simulink model "MODEL_SS_withSCCandRL_Emily_Sim_v1"  (R2024b)
settings: Solver=VariableStepAuto  StartTime=0.0  StopTime=80  RelTol=1e-3
PostLoadFcn:
  | Cconst = 0.15915494327;
  | Kp = [76; 141.7; 139.6; 114.2]*Cconst/60;
  | Tp = [14.4; 19.1; 9.39; 9.12];
  | Tg = 0.38*ones(4,1);
  | R = 3/60*ones(4,1);
  | Bagc = [0.416; 0.377; 0.378; 0.388]*60;
  | Kagc = [0.75; 0.25; 0.5; 0.5]*(-0.131);
  | Kdc = ones(4,1);
  | 
  | T = zeros(4,4);
  | T(1, 2) = 0.029;
  | T(1, 3) = 0.0143;
  | T(1, 4) = 0.0099;
  | T(2, 3) = 0.0205;
  | T(3, 4) = 0.0089;
  | T = T.*(60/Cconst);
  | T = T + T';
  | 
  | % State space of system with AGC
  | % x = [Pc Pg w Ptie]
  | % u = [Pl Pdc Pi+1 Pi+2 Pi+3]
  | clear AMatrices BMatrices
  | AMatrices(4) = struct();
  | BMatrices(4) = struct();
  | for i = 1:4
  |     Amatrix = [
  |         0, 0, Kagc(i)*Bagc(i), Kagc(i)
  |         1/Tg(i), -1/Tg(i), -1/Tg(i)/R(i), 0
  |         0, Kp(i), -Tp(i), -Kp(i)
  |         0, 0, sum(T(i,:)), 0
  |     ];
  |     AMatrices(i).value = Amatrix;
  |     Bmatrix = [
  |         0,Kagc(i)*Kdc(i),0,0,0
  |         0,0,0,0,0
  |         -Kp(i),-Kp(i)*Kdc(i),0,0,0
  |         0,0,-T(i, mod(i,4)+1),-T(i, mod(i+1,4)+1),-T(i, mod(i+2,4)+1)
  |     ];
  |     BMatrices(i).value = Bmatrix;
  | end
  | 
  | % Safety Critical Controller system
  | % The input to this system also include the AGC inputs Pc
  | % x = [Pg w Ptie]1,2,3,4
  | % u = [Pc Pl Pdc]1,2,3,4
  | 
  | Ascc = [
  |     AMatrices(1).value(2:4, 2:4), ...
  |     [zeros(3,1), BMatrices(1).value(2:4,3), zeros(3,1)], ...
  |     [zeros(3,1), BMatrices(1).value(2:4,4), zeros(3,1)], ...
  |     [zeros(3,1), BMatrices(1).value(2:4,5), zeros(3,1)]
  | 
  |     [zeros(3,1), BMatrices(2).value(2:4,3), zeros(3,1)], ...
  |     AMatrices(2).value(2:4, 2:4), ...
  |     [zeros(3,1), BMatrices(2).value(2:4,4), zeros(3,1)], ...
  |     [zeros(3,1), BMatrices(2).value(2:4,5), zeros(3,1)]
  | 
  |     [zeros(3,1), BMatrices(3).value(2:4,3), zeros(3,1)], ...
  |     [zeros(3,1), BMatrices(3).value(2:4,4), zeros(3,1)], ...
  |     AMatrices(3).value(2:4, 2:4), ...
  |     [zeros(3,1), BMatrices(3).value(2:4,5), zeros(3,1)]
  | 
  |     [zeros(3,1), BMatrices(4).value(2:4,3), zeros(3,1)], ...
  |     [zeros(3,1), BMatrices(4).value(2:4,4), zeros(3,1)], ...
  |     [zeros(3,1), BMatrices(4).value(2:4,5), zeros(3,1)], ...
  |     AMatrices(4).value(2:4, 2:4)
  | ];
  | 
  | Bscc = [
  |     AMatrices(1).value(2:4, 1), ...
  |     BMatrices(1).value(2:4, 1:2), ...
  |     zeros(3, 9)
  | 
  |     zeros(3,3), ...
  |     AMatrices(2).value(2:4, 1), ...
  |     BMatrices(2).value(2:4, 1:2), ...
  |     zeros(3,6)
  | 
  |     zeros(3,6), ...
  |     AMatrices(3).value(2:4, 1), ...
  |     BMatrices(3).value(2:4, 1:2), ...
  |     zeros(3,3)
  | 
  |     zeros(3,9), ...
  |     AMatrices(4).value(2:4, 1), ...
  |     BMatrices(4).value(2:4, 1:2)
  | ];
  | 
  | C = zeros(4,12);
  | C(1,2) = 1; C(2,5) = 1; C(3,8) = 1; C(4,11) = 1; % extracting the frequencies
libraries: dspsrcs4 x2, rllib x1
settings Model: Creator=amrmo  LastModifiedBy=emily

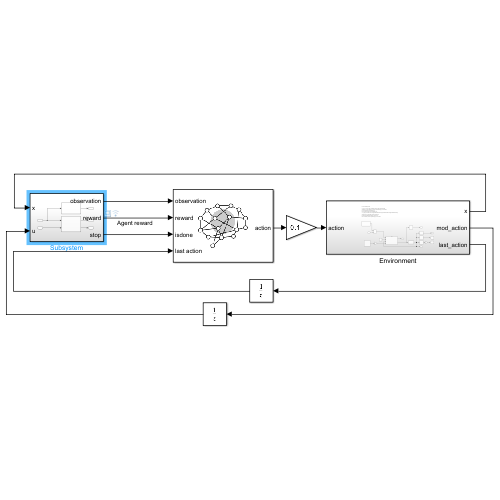
[thumbnail: Simulink's stored preview of the top-level diagram]
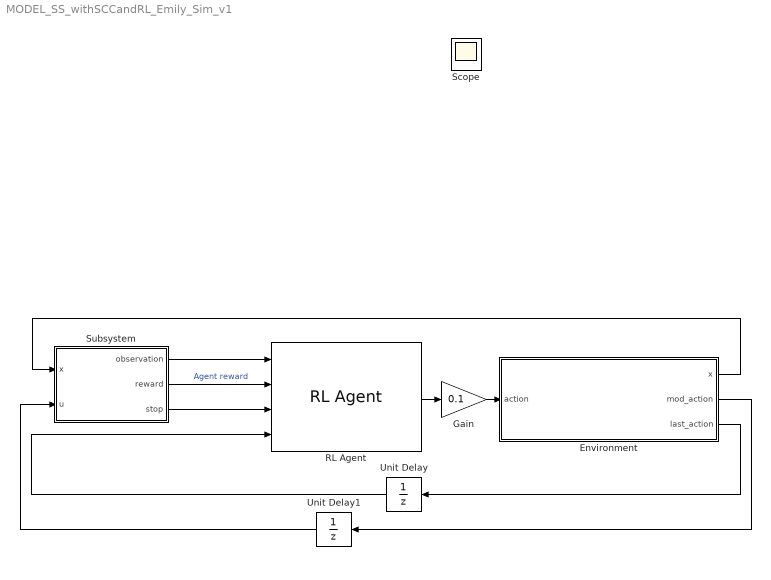
== system MODEL_SS_withSCCandRL_Emily_Sim_v1 ==
  Environment : Subsystem
  Gain : Gain  Gain=0.1
  RL Agent : rllib/RL Agent  Agent=agent  ExternalActionAsInput=off  ProvideLastAction=on  ProvideCumRwd=off  TreatAsDirectFeedthrough=on  UseStrictObservationDataTypes=off
  Subsystem : Subsystem
  Unit Delay : UnitDelay  SampleTime=-1  HasFrameUpgradeWarning=on
  Unit Delay1 : UnitDelay  SampleTime=-1  HasFrameUpgradeWarning=on
  Scope : Scope
  wires:
  RL Agent/1 -> Gain/1
  Environment/3(last_action) -> Unit Delay/1
  Environment/1(x) -> Subsystem/1(x)
  Subsystem/3(stop) -> RL Agent/3
  Subsystem/2(reward) -> RL Agent/2  "Agent reward"
  Subsystem/1(observation) -> RL Agent/1
  Unit Delay/1 -> RL Agent/4
  Gain/1 -> Environment/1(action)
  Environment/2(mod_action) -> Unit Delay1/1
  Unit Delay1/1 -> Subsystem/2(u)

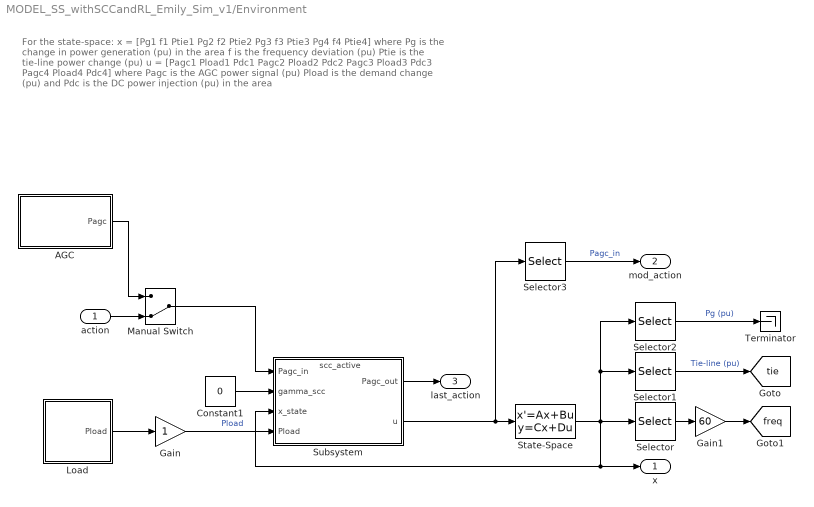
== system MODEL_SS_withSCCandRL_Emily_Sim_v1/Environment ==
  note: For the state-space:
      | x = [Pg1 f1 Ptie1 Pg2 f2 Ptie2 Pg3 f3 Ptie3 Pg4 f4 Ptie4]
      | where Pg is the change in power generation (pu) in the area
      | f is the frequency deviation (pu)
      | Ptie is the tie-line power change (pu)
      | u = [Pagc1 Pload1 Pdc1 Pagc2 Pload2 Pdc2 Pagc3 Pload3 Pdc3 Pagc4 Pload4 Pdc4]
      | where Pagc is the AGC power signal (pu)
      | Pload is the demand change (pu) and
      | Pdc is the DC power injection (pu) in the area
  action : Inport
  AGC : Subsystem
  Constant1 : Constant  Value=0
  Gain : Gain
  Gain1 : Gain  Gain=60
  Load : Subsystem
  Manual Switch : ManualSwitch  CurrentSetting=0
  Selector : Selector  InputPortWidth=12  IndexOptions=Index vector (dialog)  Indices=[2, 5, 8, 11]  OutputSizes=1
  Selector1 : Selector  InputPortWidth=12  IndexOptions=Index vector (dialog)  Indices=[3, 6, 9, 12]  OutputSizes=1
  Selector2 : Selector  InputPortWidth=12  IndexOptions=Index vector (dialog)  Indices=[1, 4, 7, 10]  OutputSizes=1
  Selector3 : Selector  InputPortWidth=12  IndexOptions=Index vector (dialog)  Indices=[1, 4, 7, 10]  OutputSizes=1
  State-Space : StateSpace  A=Ascc  B=Bscc  C=eye(size(Ascc,1))  D=zeros(size(Ascc,1), size(Bscc,2))  InitialCondition=0
  Subsystem : Subsystem
      settings: PortSchema="{\"entries\":[{\"content\":{\"sides\":[{\"content\":{\"connectorIds\":[\"In1\",\"In2\",\"In3\",\"In4\"]},\"type\":\"ConnectorPlacement.EquallySpacedRectSide\",\"uuid\":\"8ad80700-b038-40e4-a204-e695f2c66b8e\"},{\"content\":{\"connectorIds\":[\"Out1\",\"Out2\"],\"side\":\"RIGHT\"},\"type\":\"ConnectorPlacement.EquallySpacedRectSide\",\"uuid\":\"cb352c72-7f98-48f9-8295-4293ff514381\"},{\"content\":{\"connectorIds\":[\"Out3\"],\"side\":\"TOP\"},\"type\":\"ConnectorPlacement.EquallySpacedRectSide\",\"uuid\":\"f93a8a53-617b-4279-a8c2-a1411ef0bdbe\"}]},\"type\":\"ConnectorPlacement.EquallySpacedConnector\",\"uuid\":\"ea4f9763-0230-4afd-86db-2092d4b33ed4\"}],\"packageUris\":[\"http://schema.mathworks.com/mf0/Connector/R2020b\"],\"version\":\"1.0\"}"
  Terminator : Terminator
  x : Outport
  mod_action : Outport  Port=2
  last_action : Outport  Port=3
  tag scope: freq=global, tie=global
  wires:
  Subsystem/2(u) -> Selector3/1, State-Space/1
  Load/1(Pload) -> Gain/1
  Constant1/1 -> Subsystem/2(gamma_scc)
  Gain1/1 -> [freq]
  AGC/1(Pagc) -> Manual Switch/1
  Selector2/1 -> Terminator/1  "Pg (pu)"
  Selector/1 -> Gain1/1
  State-Space/1 -> Selector2/1, Selector1/1, x/1, Subsystem/3(x_state), Selector/1
  Gain/1 -> Subsystem/4(Pload)  "Pload"
  Manual Switch/1 -> Subsystem/1(Pagc_in)
  Selector1/1 -> [tie]  "Tie-line (pu)"
  action/1 -> Manual Switch/2
  Subsystem/1(Pagc_out) -> last_action/1
  Selector3/1 -> mod_action/1  "Pagc_in"

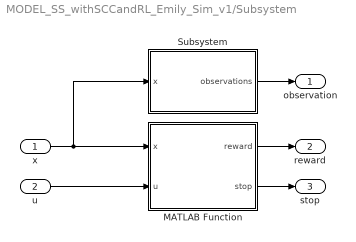
== system MODEL_SS_withSCCandRL_Emily_Sim_v1/Subsystem ==
  x : Inport
  u : Inport  Port=2
  MATLAB Function : MATLAB Function  TreatAsAtomicUnit=on
  Subsystem : Subsystem
  observation : Outport
  reward : Outport  Port=2
  stop : Outport  Port=3
  wires:
  x/1 -> Subsystem/1(x), MATLAB Function/1(x)
  Subsystem/1(observations) -> observation/1
  MATLAB Function/1(reward) -> reward/1
  MATLAB Function/2(stop) -> stop/1
  u/1 -> MATLAB Function/2(u)

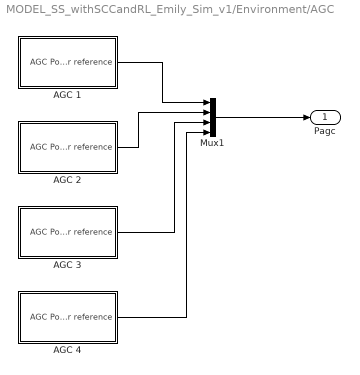
== system MODEL_SS_withSCCandRL_Emily_Sim_v1/Environment/AGC ==
  AGC 1 : Subsystem
  AGC 2 : Subsystem
  AGC 3 : Subsystem
  AGC 4 : Subsystem
  Mux1 : Mux
  Pagc : Outport
  wires:
  AGC 3/1(AGC Power reference) -> Mux1/3
  AGC 4/1(AGC Power reference) -> Mux1/4
  AGC 1/1(AGC Power reference) -> Mux1/1
  AGC 2/1(AGC Power reference) -> Mux1/2
  Mux1/1 -> Pagc/1

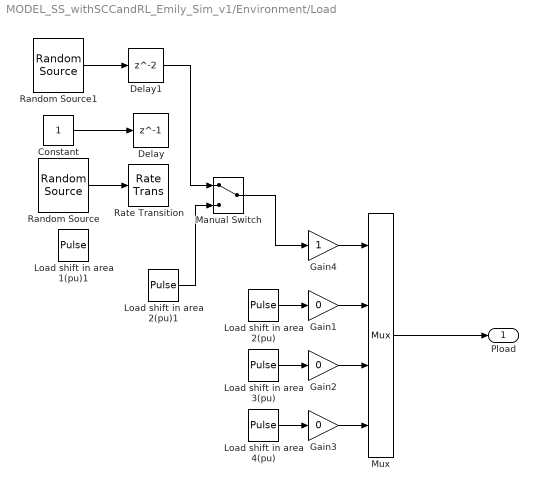
== system MODEL_SS_withSCCandRL_Emily_Sim_v1/Environment/Load ==
  Constant : Constant
  Delay : Delay  DelayLength=1  InitialCondition=0
  Delay1 : Delay  InitialCondition=0
  Gain1 : Gain  Gain=0
  Gain2 : Gain  Gain=0
  Gain3 : Gain  Gain=0
  Gain4 : Gain
  Load shift in area 1(pu)1 : DiscretePulseGenerator  PulseType=Time based  Amplitude=0.05  Period=80  PulseWidth=10  PhaseDelay=10
  Load shift in area 2(pu) : DiscretePulseGenerator  PulseType=Time based  Amplitude=0.2  Period=2*pi/2.5  PulseWidth=40
  Load shift in area 2(pu)1 : DiscretePulseGenerator  PulseType=Time based  Amplitude=0.05  Period=2*pi/2.5  PulseWidth=40
  Load shift in area 3(pu) : DiscretePulseGenerator  PulseType=Time based  Amplitude=0  Period=10  PulseWidth=5
  Load shift in area 4(pu) : DiscretePulseGenerator  PulseType=Time based  Amplitude=0  Period=10  PulseWidth=5
  Manual Switch : ManualSwitch
  Mux : Mux
  Random Source : dspsrcs4/Random Source  SrcType=Uniform  MinVal=0  MaxVal=.1  MeanVal=0  VarVal=1  RepMode=Not repeatable  rawSeed=1  IsInherit=off  SampTime=40  SampFrame=1  OutComplex=Real  DataType=double  SimulateUsing=Interpreted execution
  Random Source1 : dspsrcs4/Random Source  SrcType=Uniform  MinVal=-.05  MaxVal=0.05  MeanVal=0  VarVal=1  RepMode=Specify seed  rawSeed=1  IsInherit=off  SampTime=10  SampFrame=1  OutComplex=Real  DataType=double  SimulateUsing=Interpreted execution
  Rate Transition : RateTransition
  Pload : Outport
  wires:
  Load shift in area 4(pu)/1 -> Gain3/1
  Load shift in area 2(pu)/1 -> Gain1/1
  Load shift in area 3(pu)/1 -> Gain2/1
  Mux/1 -> Pload/1
  Gain1/1 -> Mux/2
  Gain2/1 -> Mux/3
  Gain3/1 -> Mux/4
  Gain4/1 -> Mux/1
  Manual Switch/1 -> Gain4/1
  Random Source/1 -> Rate Transition/1
  Constant/1 -> Delay/1
  Load shift in area 2(pu)1/1 -> Manual Switch/2
  Random Source1/1 -> Delay1/1
  Delay1/1 -> Manual Switch/1

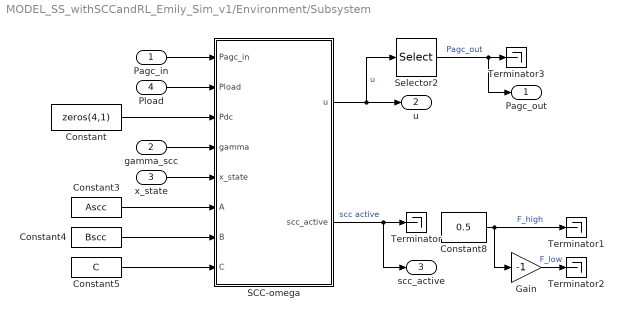
== system MODEL_SS_withSCCandRL_Emily_Sim_v1/Environment/Subsystem ==
  Pagc_in : Inport
  gamma_scc : Inport  Port=2
  x_state : Inport  Port=3
  Pload : Inport  Port=4
  Constant : Constant  Value=zeros(4,1)
  Constant3 : Constant  Value=Ascc
  Constant4 : Constant  Value=Bscc
  Constant5 : Constant  Value=C
  Constant8 : Constant  Value=0.5
  Gain : Gain  Gain=-1
  SCC-omega : MATLAB Function  TreatAsAtomicUnit=on
  Selector2 : Selector  InputPortWidth=12  IndexOptions=Index vector (dialog)  Indices=[1 4 7 10]  OutputSizes=1
  Terminator{,1..3} (4 alike) : Terminator
  Pagc_out : Outport
  u : Outport  Port=2
  scc_active : Outport  Port=3
  wires:
  Pload/1 -> SCC-omega/2(Pload)
  Constant5/1 -> SCC-omega/8(C)
  Constant3/1 -> SCC-omega/6(A)
  Constant/1 -> SCC-omega/3(Pdc)
  SCC-omega/1(u) -> u/1, Selector2/1  "u"
  Selector2/1 -> Pagc_out/1, Terminator3/1  "Pagc_out"
  Constant4/1 -> SCC-omega/7(B)
  x_state/1 -> SCC-omega/5(x_state)
  gamma_scc/1 -> SCC-omega/4(gamma)
  Pagc_in/1 -> SCC-omega/1(Pagc_in)
  SCC-omega/2(scc_active) -> scc_active/1, Terminator/1  "scc active"
  Constant8/1 -> Terminator1/1, Gain/1  "F_high"
  Gain/1 -> Terminator2/1  "F_low"

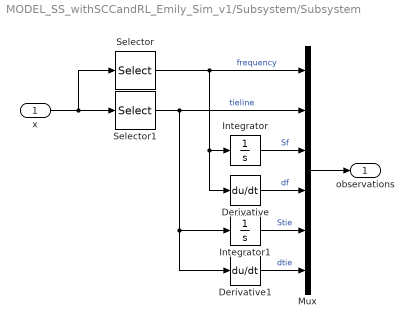
== system MODEL_SS_withSCCandRL_Emily_Sim_v1/Subsystem/Subsystem ==
  x : Inport
  Derivative : Derivative
  Derivative1 : Derivative
  Integrator : Integrator
  Integrator1 : Integrator
  Mux : Mux  Inputs=6
  Selector : Selector  InputPortWidth=12  IndexOptions=Index vector (dialog)  Indices=[2,5,8,11]  OutputSizes=1
  Selector1 : Selector  InputPortWidth=12  IndexOptions=Index vector (dialog)  Indices=[3 6 9 12]  OutputSizes=1
  observations : Outport
  wires:
  Derivative1/1 -> Mux/6  "dtie"
  Derivative/1 -> Mux/4  "df"
  Selector/1 -> Derivative/1, Integrator/1, Mux/1  "frequency"
  Selector1/1 -> Derivative1/1, Integrator1/1, Mux/2  "tieline"
  x/1 -> Selector1/1, Selector/1
  Integrator/1 -> Mux/3  "Sf"
  Integrator1/1 -> Mux/5  "Stie"
  Mux/1 -> observations/1

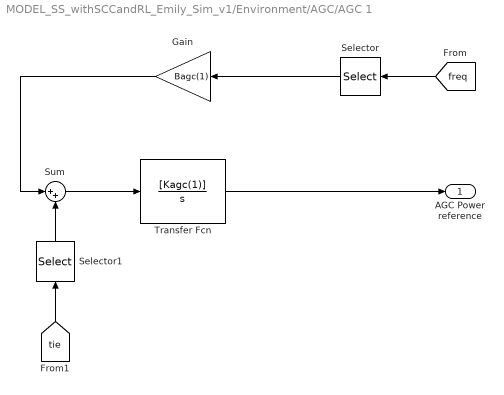
== system MODEL_SS_withSCCandRL_Emily_Sim_v1/Environment/AGC/AGC 1 ==
  Gain : Gain  Gain=Bagc(1)
  Selector : Selector  InputPortWidth=4  IndexOptions=Index vector (dialog)  Indices=[1]  OutputSizes=1
  Selector1 : Selector  InputPortWidth=4  IndexOptions=Index vector (dialog)  Indices=[1]  OutputSizes=1
  Sum : Sum  Inputs=|++
  Transfer Fcn : TransferFcn  Numerator=[Kagc(1)]  Denominator=[1 0]
  AGC Power reference : Outport
  wires:
  Transfer Fcn/1 -> AGC Power reference/1
  Sum/1 -> Transfer Fcn/1
  Gain/1 -> Sum/1
  Selector/1 -> Gain/1
  Selector1/1 -> Sum/2
  [freq] -> Selector/1
  [tie] -> Selector1/1

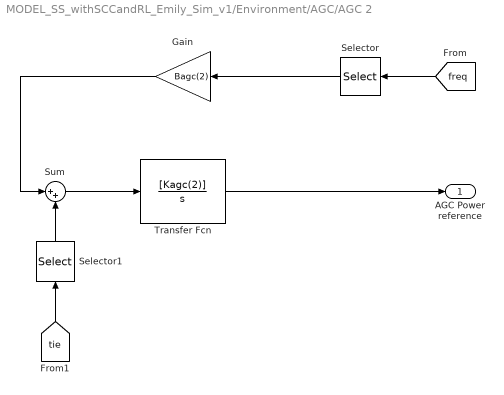
== system MODEL_SS_withSCCandRL_Emily_Sim_v1/Environment/AGC/AGC 2 ==
  Gain : Gain  Gain=Bagc(2)
  Selector : Selector  InputPortWidth=4  IndexOptions=Index vector (dialog)  Indices=[2]  OutputSizes=1
  Selector1 : Selector  InputPortWidth=4  IndexOptions=Index vector (dialog)  Indices=[2]  OutputSizes=1
  Sum : Sum  Inputs=|++
  Transfer Fcn : TransferFcn  Numerator=[Kagc(2)]  Denominator=[1 0]
  AGC Power reference : Outport
  wires:
  Transfer Fcn/1 -> AGC Power reference/1
  Sum/1 -> Transfer Fcn/1
  Gain/1 -> Sum/1
  Selector/1 -> Gain/1
  Selector1/1 -> Sum/2
  [freq] -> Selector/1
  [tie] -> Selector1/1

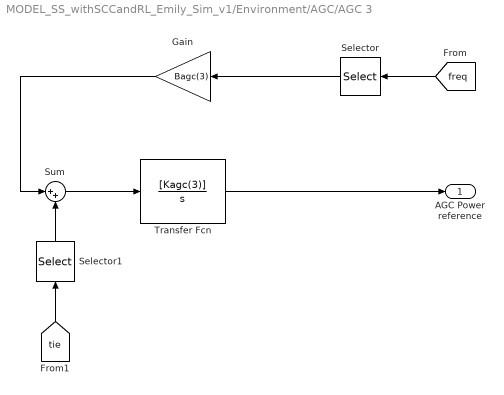
== system MODEL_SS_withSCCandRL_Emily_Sim_v1/Environment/AGC/AGC 3 ==
  Gain : Gain  Gain=Bagc(3)
  Selector : Selector  InputPortWidth=4  IndexOptions=Index vector (dialog)  Indices=[3]  OutputSizes=1
  Selector1 : Selector  InputPortWidth=4  IndexOptions=Index vector (dialog)  Indices=[3]  OutputSizes=1
  Sum : Sum  Inputs=|++
  Transfer Fcn : TransferFcn  Numerator=[Kagc(3)]  Denominator=[1 0]
  AGC Power reference : Outport
  wires:
  Transfer Fcn/1 -> AGC Power reference/1
  Sum/1 -> Transfer Fcn/1
  Gain/1 -> Sum/1
  Selector/1 -> Gain/1
  Selector1/1 -> Sum/2
  [freq] -> Selector/1
  [tie] -> Selector1/1

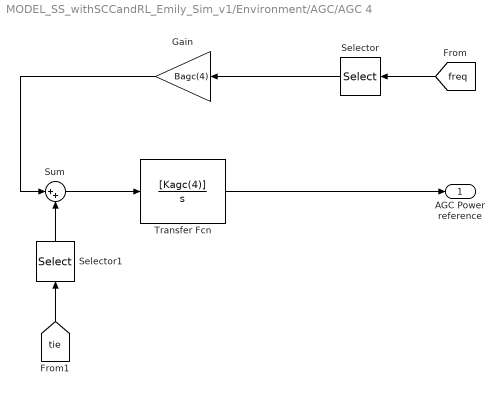
== system MODEL_SS_withSCCandRL_Emily_Sim_v1/Environment/AGC/AGC 4 ==
  Gain : Gain  Gain=Bagc(4)
  Selector : Selector  InputPortWidth=4  IndexOptions=Index vector (dialog)  Indices=[4]  OutputSizes=1
  Selector1 : Selector  InputPortWidth=4  IndexOptions=Index vector (dialog)  Indices=[4]  OutputSizes=1
  Sum : Sum  Inputs=|++
  Transfer Fcn : TransferFcn  Numerator=[Kagc(4)]  Denominator=[1 0]
  AGC Power reference : Outport
  wires:
  Transfer Fcn/1 -> AGC Power reference/1
  Sum/1 -> Transfer Fcn/1
  Gain/1 -> Sum/1
  Selector/1 -> Gain/1
  Selector1/1 -> Sum/2
  [freq] -> Selector/1
  [tie] -> Selector1/1

== matlab function MODEL_SS_withSCCandRL_Emily_Sim_v1/Subsystem/MATLAB Function ==
  data: x input; reward output; stop output; u input
function [reward, stop] = fcn(x, u)
%#codegen
    frequency = reshape(x([2,5,8,11]), [4,1]);
    tie_line = reshape(x([3,6,9,12]), [4,1]);
    u = reshape(u, [4,1]);
    
    F = 0.5/60; % upper frequency limit

    Q1 = eye(4)*(60/0.4)^2;
    Q2 = eye(4)*(1/0.1)^2;
    R = eye(4)*(1/0.1)^2;

    stop = any(abs(frequency) > F);
    reward = - frequency'*Q1*frequency - tie_line'*Q2*tie_line ...
        - 0.1*u'*R*u - 1E3*stop;
end

== matlab function MODEL_SS_withSCCandRL_Emily_Sim_v1/Environment/Subsystem/SCC-omega ==
  data: Pagc_in input; u output; Pload input; Pdc input; gamma input; scc_active output; x_state input; A input; B input; C input
function [u, scc_active] = fcn(Pagc_in, Pload, Pdc, gamma , x_state, ...
    A, B, C)
    %{
        INPUTS: 
        - Pagc_in: float(4,1): is the agc control signal (pu) to each of areas 1, 2, 3, 4
        - Pload: float(4,1): is the load change (pu) in areas 1, 2, 3, 4
        - Pdc: float(4,1): is the dc power injection (pu) to areas 1, 2, 3, 4
        - x_state: float(12,1): is the state of the system [Pg (pu), frequency (pu), Ptie
        (pu)]1,2,3,4
        
        - alpha_scc: float(1,1): is the alpha parameter of the safety-critical controller.
        alpha_scc = 0 deactivates the safety critical controller.
        Lower alpha_scc makes the safety critical controller less relaxed.
        
        OUTPUTS:
        - u: float(12,1): is the input to the system consisting of [Pagc (pu), Pload (pu), 
        Pds (pu)]1,2,3,4
        - scc_active \in {0,1} is a boolean for whether the safety critical controller
        was activated or not.
        
    %}
    coder.extrinsic('safety_critical_controller');
    u = zeros(12,1);
    scc_active = 0;
    [u, scc_active] = safety_critical_controller(Pagc_in, Pload, Pdc, gamma , x_state, ...
    A, B, C);
end
